simulink model "pil_tmu_am13x"  (R2025b)
settings: Solver=FixedStepAuto  StartTime=0.0  StopTime=1  RelTol=1e-3  EnableMultiTasking=on
libraries: simulink x1
settings Model: SimulationMode=processor-in-the-loop (pil)  CodeVerificationMode=processor-in-the-loop (pil)  Creator=a1255762  LastModifiedBy=a1255762
settings OptimizationCC: DefaultParameterBehavior=Inlined  DefaultUnderspecifiedDataType=single  EnhancedBackFolding=on  ZeroExternalMemoryAtStartup=off  ZeroInternalMemoryAtStartup=off  MaxStackSize=64  OptimizeBlockOrder=speed  DifferentSizesBufferReuse=on  OptimizationCustomize=off  EfficientTunableParamExpr=on
settings DebuggingCC: ParameterPrecisionLossMsg=none  ParameterTunabilityLossMsg=error
settings HardwareCC: ProdBitPerPointer=32.0  ProdBitPerSizeT=32.0  ProdBitPerPtrDiffT=32.0  ProdLargestAtomicInteger=Long  ProdLargestAtomicFloat=Double  ProdWordSize=32.0  ProdLongLongMode=on  ProdHWDeviceType=ARM Compatible->ARM Cortex
settings SFSimCC: MATLABDynamicMemAlloc=off
settings RTWCC: SystemTargetFile=ert.tlc  HardwareBoard=AM13E230x  GenCodeOnly=on  TemplateMakefile=ert_default_tmf  GenerateReport=on  Toolchain=TI ARM Clang Compiler AM13x | gmake  BuildConfiguration=Faster Runs  IncludeHyperlinkInReport=on  LaunchReport=on  CodeExecutionProfiling=on  CodeProfilingInstrumentation=detailed  GenerateTraceInfo=on  GenerateCodeReplacementReport=on  Description=Embedded Coder
settings CodeAppCC: ForceParamTrailComments=on  IgnoreCustomStorageClasses=off  MaxIdLength=256.0  OperatorAnnotations=on  SimulinkDataObjDesc=on  SFDataObjDesc=on  InsertBlockDesc=on
settings ERTTargetCC: ExtModeTransport=3.0  ExtModeStaticAlloc=on  ExtModeMexFile=ext_xcp  ExtModeIntrfLevel=Level2 - Open  InlinedParameterPlacement=Hierarchical  ERTCustomFileTemplate=AM13x_codertarget_file_process.tlc  CodeReplacementLibrary=AM13x_TMU

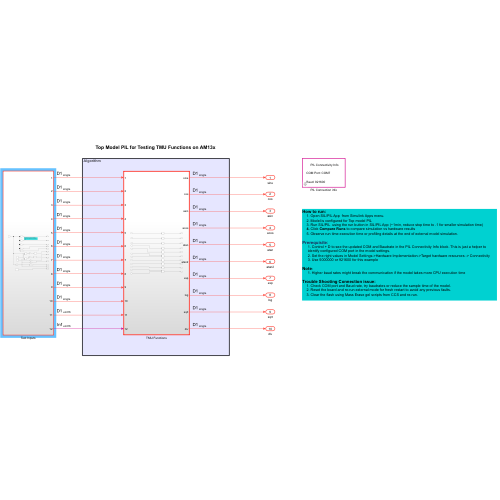
[thumbnail: Simulink's stored preview of the top-level diagram]
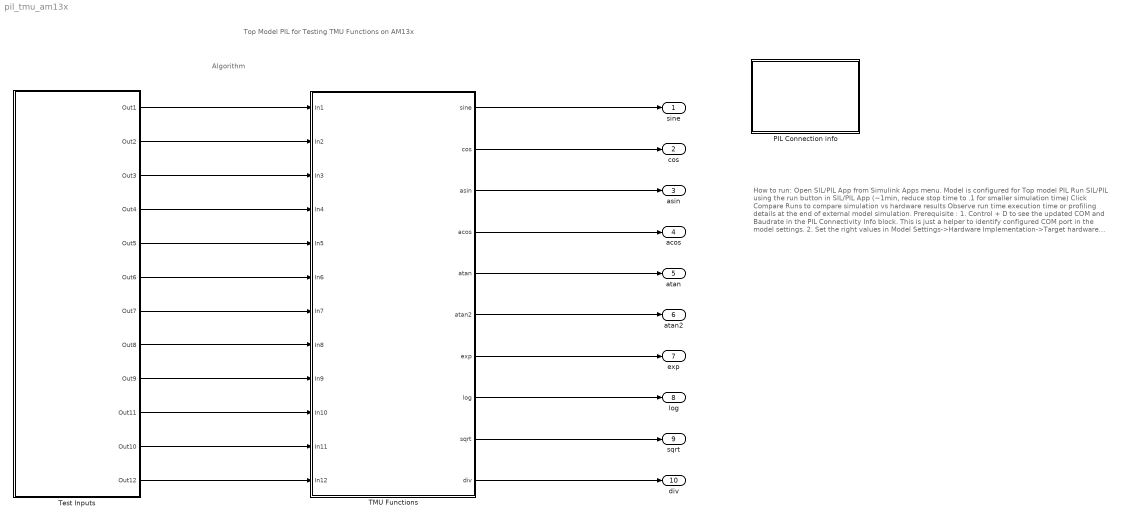
== system pil_tmu_am13x ==
  note: Algorithm
  note: How to run:
      | Open SIL/PIL App from Simulink Apps menu.
      | Model is configured for Top model PIL
      | Run SIL/PIL using the run button in SIL/PIL App (~1min, reduce stop time to .1 for smaller simulation time)
      | Click Compare Runs to compare simulation vs hardware results
      | Observe run time execution time or profiling details at the end of external model simulation.
      |
      | Prerequisite :
      | 1. Control + D to see the updated COM and Baudrate in the PIL Connectivity Info block. This is just a helper to identify configured COM port in the model settings.
      | 2. Set the right values in Model Settings->Hardware Implementation->Target hardware resources -> Connectivity
      | 3. Use 5000000 or 921600 for this example
      |
      | Note :
      | 1. Higher baud rates might break the communication if the model takes more CPU execution time
      |
      | Trouble Shooting Connection issue:
      | Check COM port and Baud rate, try baudrates or reduce the sample time of the model.
      | Reset the board and re-run external mode for fresh restart to avoid any previous faults.
      | Clear the flash using Mass Erase gel scripts from CCS and re-run.
  note: Top Model PIL for Testing TMU Functions on AM13x
  PIL Connection info : Subsystem  mask{Parameter1=|}
      mask Parameter1=|
      | codertarget.data.setParameterValue(bdroot, 'Connection.Serialport', 'COM3')
      | codertarget.data.setParameterValue(bdroot, 'Connection.Baud', '5000000')
      mask prompts: Parameter1 "Change programmatically"
      mask Display:
      | % Update mask parameters with current values when opened
      | 
      | pilData = codertarget.data.getParameterValue(bdroot, 'Connection');
      | 
      | 
      | % Use text() function with specific positioning
      | text(0.2, 0.8, 'PIL Connectivity Info', 'HorizontalAlignment', 'left');
      | text(0.1, 0.5, ['COM Port: ' pilData.Serialport], 'HorizontalAlignment', 'left');
      | text(0.1, 0.2, ['Baud: ' pilData.Baud], 'HorizontalAlignment', 'left');
  TMU Functions : Subsystem  TreatAsAtomicUnit=on
      settings: RTWSystemCode=Nonreusable function
  Test Inputs : Subsystem
  sine : Outport
  cos : Outport  Port=2
  asin : Outport  Port=3
  acos : Outport  Port=4
  atan : Outport  Port=5
  atan2 : Outport  Port=6
  exp : Outport  Port=7
  log : Outport  Port=8
  sqrt : Outport  Port=9
  div : Outport  Port=10
  wires:
  TMU Functions/1(sine) -> sine/1
  TMU Functions/10(div) -> div/1
  TMU Functions/2(cos) -> cos/1
  TMU Functions/9(sqrt) -> sqrt/1
  TMU Functions/8(log) -> log/1
  TMU Functions/3(asin) -> asin/1
  TMU Functions/7(exp) -> exp/1
  TMU Functions/5(atan) -> atan/1
  TMU Functions/6(atan2) -> atan2/1
  TMU Functions/4(acos) -> acos/1
  Test Inputs/1(Out1) -> TMU Functions/1(In1)
  Test Inputs/2(Out2) -> TMU Functions/2(In2)
  Test Inputs/3(Out3) -> TMU Functions/3(In3)
  Test Inputs/4(Out4) -> TMU Functions/4(In4)
  Test Inputs/5(Out5) -> TMU Functions/5(In5)
  Test Inputs/6(Out6) -> TMU Functions/6(In6)
  Test Inputs/7(Out7) -> TMU Functions/7(In7)
  Test Inputs/8(Out8) -> TMU Functions/8(In8)
  Test Inputs/9(Out9) -> TMU Functions/9(In9)
  Test Inputs/12(Out12) -> TMU Functions/12(In12)
  Test Inputs/10(Out11) -> TMU Functions/10(In10)
  Test Inputs/11(Out10) -> TMU Functions/11(In11)

== system pil_tmu_am13x/PIL Connection info ==

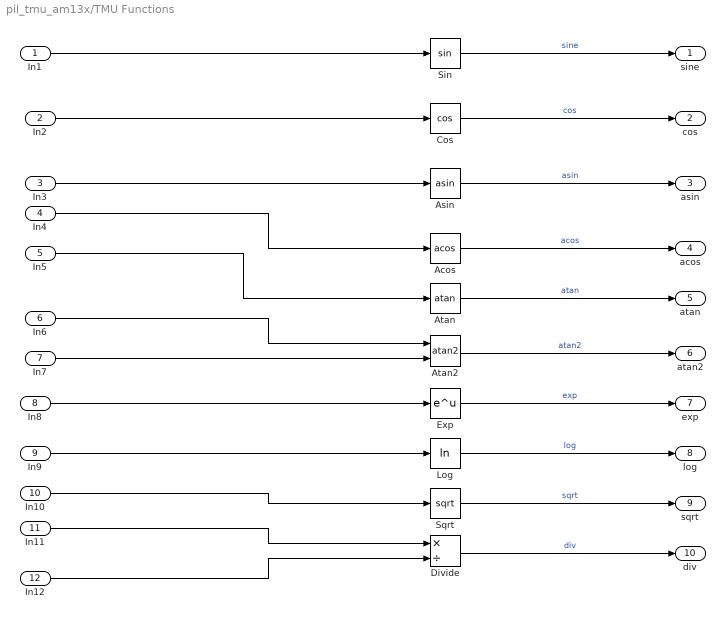
== system pil_tmu_am13x/TMU Functions ==
  In1 : Inport
  In2 : Inport  Port=2
  In3 : Inport  Port=3
  In4 : Inport  Port=4
  In5 : Inport  Port=5
  In6 : Inport  Port=6
  In7 : Inport  Port=7
  In8 : Inport  Port=8
  In9 : Inport  Port=9
  In10 : Inport  Port=10
  In11 : Inport  Port=11
  In12 : Inport  Port=12
  Acos : Trigonometry  Operator=acos
  Asin : Trigonometry  Operator=asin
  Atan : Trigonometry  Operator=atan
  Atan2 : Trigonometry  Operator=atan2
  Cos : Trigonometry  Operator=cos
  Divide : Product  Inputs=*/  OutDataTypeStr=single
  Exp : Math
  Log : Math  Operator=log
  Sin : Trigonometry
  Sqrt : Sqrt
  sine : Outport
  cos : Outport  Port=2
  asin : Outport  Port=3
  acos : Outport  Port=4
  atan : Outport  Port=5
  atan2 : Outport  Port=6
  exp : Outport  Port=7
  log : Outport  Port=8
  sqrt : Outport  Port=9
  div : Outport  Port=10
  wires:
  Atan2/1 -> atan2/1  "atan2"
  In2/1 -> Cos/1
  In8/1 -> Exp/1
  In9/1 -> Log/1
  Sqrt/1 -> sqrt/1  "sqrt"
  Asin/1 -> asin/1  "asin"
  In4/1 -> Acos/1
  Sin/1 -> sine/1  "sine"
  Acos/1 -> acos/1  "acos"
  Log/1 -> log/1  "log"
  Divide/1 -> div/1  "div"
  In3/1 -> Asin/1
  Exp/1 -> exp/1  "exp"
  In7/1 -> Atan2/2
  In6/1 -> Atan2/1
  In1/1 -> Sin/1
  Atan/1 -> atan/1  "atan"
  Cos/1 -> cos/1  "cos"
  In12/1 -> Divide/2
  In10/1 -> Sqrt/1
  In11/1 -> Divide/1
  In5/1 -> Atan/1

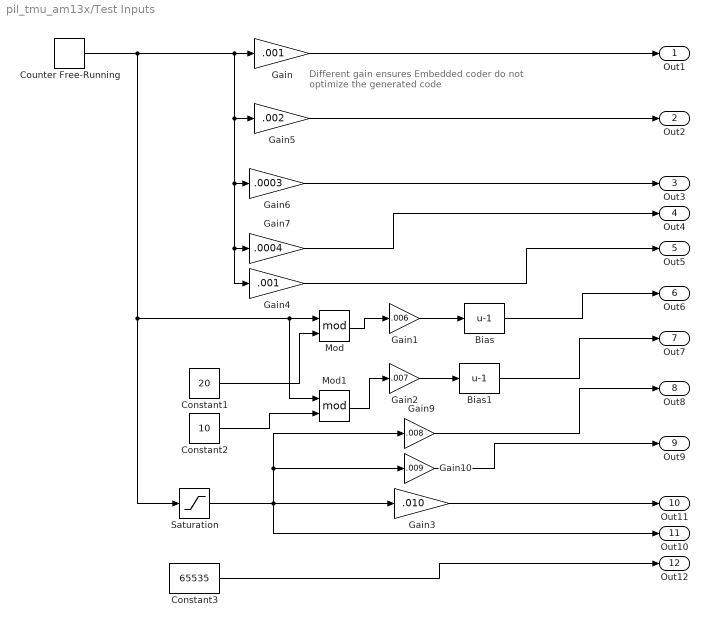
== system pil_tmu_am13x/Test Inputs ==
  note: Different gain ensures Embedded coder do not optimize the generated code
  Bias : Bias  Bias=-1  SaturateOnIntegerOverflow=off
  Bias1 : Bias  Bias=-1  SaturateOnIntegerOverflow=off
  Constant1 : Constant  Value=20  OutDataTypeStr=uint16
  Constant2 : Constant  Value=10  OutDataTypeStr=uint16
  Constant3 : Constant  Value=65535  OutDataTypeStr=uint16
  Counter Free-Running : simulink/Sources/Counter Free-Running  NumBits=16  tsamp=.001
  Gain : Gain  Gain=.001  OutDataTypeStr=single
  Gain1 : Gain  Gain=.006  OutDataTypeStr=single
  Gain10 : Gain  Gain=.009  OutDataTypeStr=single
  Gain2 : Gain  Gain=.007  OutDataTypeStr=single
  Gain3 : Gain  Gain=.010  OutDataTypeStr=single
  Gain4 : Gain  Gain=.001  OutDataTypeStr=single
  Gain5 : Gain  Gain=.002  OutDataTypeStr=single
  Gain6 : Gain  Gain=.0003  OutDataTypeStr=single
  Gain7 : Gain  Gain=.0004  OutDataTypeStr=single
  Gain9 : Gain  Gain=.008  OutDataTypeStr=single
  Mod : Math  Operator=mod
  Mod1 : Math  Operator=mod
  Saturation : Saturate  UpperLimit=65535  LowerLimit=1
  Out1 : Outport
  Out2 : Outport  Port=2
  Out3 : Outport  Port=3
  Out4 : Outport  Port=4
  Out5 : Outport  Port=5
  Out6 : Outport  Port=6
  Out7 : Outport  Port=7
  Out8 : Outport  Port=8
  Out9 : Outport  Port=9
  Out11 : Outport  Port=10
  Out10 : Outport  Port=11
  Out12 : Outport  Port=12
  wires:
  Bias1/1 -> Out7/1
  Counter Free-Running/1 -> Saturation/1, Mod/1, Mod1/1, Gain4/1, Gain7/1, Gain6/1, Gain5/1, Gain/1
  Saturation/1 -> Gain10/1, Gain9/1, Out10/1, Gain3/1
  Gain9/1 -> Out8/1
  Constant3/1 -> Out12/1
  Mod1/1 -> Gain2/1
  Gain1/1 -> Bias/1
  Gain3/1 -> Out11/1
  Mod/1 -> Gain1/1
  Constant2/1 -> Mod1/2
  Gain10/1 -> Out9/1
  Gain2/1 -> Bias1/1
  Gain5/1 -> Out2/1
  Gain6/1 -> Out3/1
  Constant1/1 -> Mod/2
  Gain7/1 -> Out4/1
  Bias/1 -> Out6/1
  Gain/1 -> Out1/1
  Gain4/1 -> Out5/1
